simulink model "onboard_matlab"  (Simulink 8.1)
settings: Solver=FixedStepDiscrete  SolverMode=MultiTasking  StartTime=0.0  StopTime=30  FixedStep=Sampletime.Onboard  RelTol=1e-3
PreLoadFcn:
  | InitOnboardMatlab_bus;
InitFcn:
  | InitOnboardMatlab;
undefined symbols (not defined in the file or in its folder): DiscIntNeverNeededParam, Sampletime, uart_up_p_01, uart_up_p_02, uart_up_p_10, uart_up_p_11, uart_up_p_12, uart_up_p_13, uart_up_p_14
libraries: simulink x5
CloseFcn:
  | rtwprivate ssgencode ModelCloseRequest onboard_matlab
settings Model: MinMaxOverflowLogging=MinMaxAndOverflow  Creator=Holzapfel  LastModifiedBy=Javid  TunableVars=uart_up_p_01,uart_up_p_02,uart_up_p_03,uart_up_p_04,uart_up_p_05,uart_up_p_06,uart_up_p_07,uart_up_p_08,uart_up_p_09,uart_up_p_10,uart_up_p_11,uart_up_p_12,uart_up_p_13,uart_up_p_14,uart_up_p_15,uart_up_p_16,uart_up_p_17,uart_up_p_18,uart_up_p_19,uart_up_p_20,uart_up_p_21,uart_up_p_22,uart_up_p_23,uart_up_p_24,uart_up_p_25,uart_up_p_26,uart_up_p_27,uart_up_p_28,uart_up_p_29,uart_up_p_30,uart_up_p_31,uart_up_p_32,uart_up_p_33,uart_up_p_34,uart_up_p_35,uart_up_p_36,uart_up_p_37,uart_up_p_38,uart_up_p_39,uart_up_p_40  TunableVarsStorageClass=ImportedExtern,ImportedExtern,ImportedExtern,ImportedExtern,ImportedExtern,ImportedExtern,ImportedExtern,ImportedExtern,ImportedExtern,ImportedExtern,ImportedExtern,ImportedExtern,ImportedExtern,ImportedExtern,ImportedExtern,ImportedExtern,ImportedExtern,ImportedExtern,ImportedExtern,ImportedExtern,ImportedExtern,ImportedExtern,ImportedExtern,ImportedExtern,ImportedExtern,ImportedExtern,ImportedExtern,ImportedExtern,ImportedExtern,ImportedExtern,ImportedExtern,ImportedExtern,ImportedExtern,ImportedExtern,ImportedExtern,ImportedExtern,ImportedExtern,ImportedExtern,ImportedExtern,ImportedExtern  TunableVarsTypeQualifier=,,,,,,,,,,,,,,,,,,,,,,,,,,,,,,,,,,,,,,,
settings DataIOCC: LimitDataPoints=off  SaveOutput=off  SignalLogging=off  DSMLogging=off  SaveTime=off
settings OptimizationCC: InlineParams=on  InlineInvariantSignals=on  EnableMemcpy=off  StateBitsets=on  DataBitsets=on  UseTempVars=on  ZeroExternalMemoryAtStartup=off  ZeroInternalMemoryAtStartup=off  NoFixptDivByZeroProtection=on  EfficientFloat2IntCast=on  OptimizeModelRefInitCode=on  LifeSpan=1  SimCompilerOptimization=On
settings DebuggingCC: ConsistencyChecking=error  ArrayBoundsChecking=error  SignalInfNanChecking=error  SignalRangeChecking=error  ReadBeforeWriteMsg=EnableAllAsError  WriteAfterWriteMsg=EnableAllAsError  WriteAfterReadMsg=EnableAllAsError  AlgebraicLoopMsg=error  ArtificialAlgebraicLoopMsg=error  SaveWithDisabledLinksMsg=error  SaveWithParameterizedLinksMsg=error  CheckExecutionContextPreStartOutputMsg=on  CheckExecutionContextRuntimeOutputMsg=on  BlockPriorityViolationMsg=error  MinStepSizeMsg=error  TimeAdjustmentMsg=warning  SolverPrmCheckMsg=error  InheritedTsInSrcMsg=error  DiscreteInheritContinuousMsg=error  SingleTaskRateTransMsg=error  TasksWithSamePriorityMsg=error  SigSpecEnsureSampleTimeMsg=error  CheckMatrixSingularityMsg=error  IntegerOverflowMsg=error  ParameterUnderflowMsg=warning  ParameterTunabilityLossMsg=error  UnderSpecifiedDataTypeMsg=error  UnnecessaryDatatypeConvMsg=warning  VectorMatrixConversionMsg=error  SignalLabelMismatchMsg=error  UnconnectedInputMsg=error  UnconnectedOutputMsg=error  UnconnectedLineMsg=error  SFcnCompatibilityMsg=error  UniqueDataStoreMsg=error  BusObjectLabelMismatch=error  RootOutportRequireBusObject=error  ModelReferenceIOMsg=error  ModelReferenceVersionMismatchMessage=error  ModelReferenceIOMismatchMessage=error  ModelReferenceCSMismatchMessage=error  UnknownTsInhSupMsg=error  ModelReferenceDataLoggingMessage=error  StrictBusMsg=ErrorOnBusTreatedAsVector  LoggingUnavailableSignals=none
settings HardwareCC: ProdLargestAtomicInteger=Long  ProdLargestAtomicFloat=Float  ProdIntDivRoundTo=Zero  ProdEndianess=LittleEndian  ProdHWDeviceType=ARM Compatible->ARM 7  TargetEndianess=LittleEndian  TargetHWDeviceType=ARM Compatible->ARM 7
settings SFSimCC: SimParseCustomCode=off
settings RTWCC: SystemTargetFile=ert.tlc  GenCodeOnly=on  MakeCommand=make_rtw optimized_fixed_point=1  GenerateMakefile=off  TemplateMakefile=ert_default_tmf  Description=Real-Time Workshop Embedded Coder (auto configures for optimized fixed-point code)  GenerateReport=on  ProcessScript=ert_make_rtw_hook  IncludeHyperlinkInReport=on  LaunchReport=on  GenerateTraceInfo=on
settings RTWCC: CustomHeaderCode=|
  | #undef a
  | #undef b
settings CodeAppCC: IgnoreCustomStorageClasses=off  CustomSymbolStrType=$N$R$M  InternalIdentifier=Classic
settings ERTTargetCC: CodeReplacementLibrary=ANSI_C  MultiwordLength=2048  GenerateSampleERTMain=on  IncludeMdlTerminateFcn=off  SuppressErrorStatus=on  SupportNonFinite=off  SupportComplex=off  PurelyIntegerCode=on  ExtModeTransport=1  ExtModeMexFile=ext_serial_win32_comm  InlinedParameterPlacement=NonHierarchical  ERTCustomFileTemplate=file_process.tlc  ConvertIfToSwitch=off  SuppressUnreachableDefaultCases=off

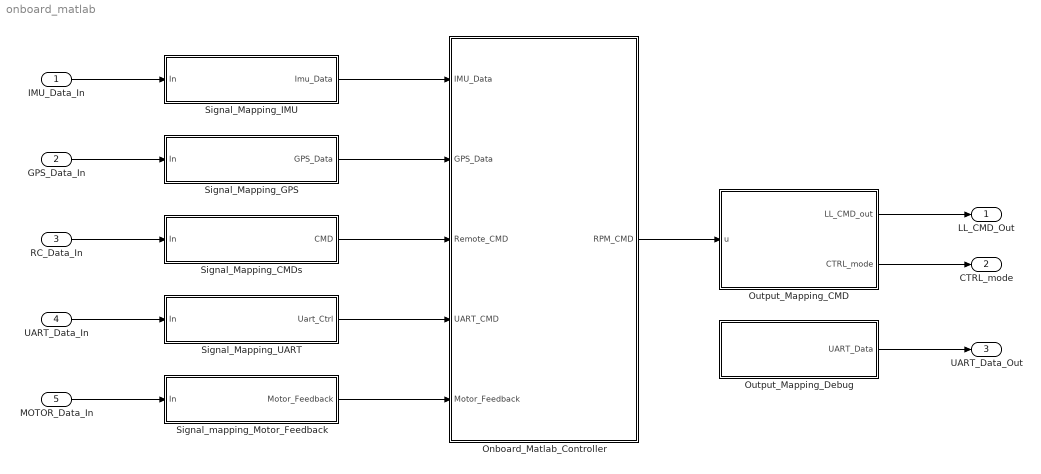
== system onboard_matlab ==
  IMU_Data_In : Inport  OutMin=-2^31  OutMax=2^31-1  OutDataTypeStr=Bus: IMU_DATA_IN  SampleTime=Sampletime.Onboard  BusOutputAsStruct=on
  GPS_Data_In : Inport  Port=2  OutMin=-2^31  OutMax=2^31-1  OutDataTypeStr=Bus: GPS_DATA_IN  SampleTime=Sampletime.Onboard  BusOutputAsStruct=on
  RC_Data_In : Inport  Port=3  OutMin=-2^15  OutMax=2^15-1  OutDataTypeStr=Bus: RC_DATA_IN  SampleTime=Sampletime.Onboard  BusOutputAsStruct=on
  UART_Data_In : Inport  Port=4  OutMin=-2^15  OutMax=2^15-1  OutDataTypeStr=Bus: UART_DATA_IN  SampleTime=Sampletime.Onboard  BusOutputAsStruct=on
  MOTOR_Data_In : Inport  Port=5  OutMin=0  OutMax=200  OutDataTypeStr=Bus: MOTOR_DATA_IN  SampleTime=Sampletime.Onboard  BusOutputAsStruct=on
  Onboard_Matlab_Controller : Subsystem  MinMaxOverflowLogging=MinMaxAndOverflow
  Output_Mapping_CMD : Subsystem
  Output_Mapping_Debug : Subsystem
  Signal_Mapping_CMDs : Subsystem
  Signal_Mapping_GPS : Subsystem
  Signal_Mapping_IMU : Subsystem
  Signal_Mapping_UART : Subsystem
  Signal_mapping_Motor_Feedback : Subsystem
  LL_CMD_Out : Outport  OutDataTypeStr=Bus: LL_CMD_OUT  SampleTime=Sampletime.Onboard  BusOutputAsStruct=on
  CTRL_mode : Outport  Port=2  OutDataTypeStr=Bus: CTRL_MODE  SampleTime=Sampletime.Onboard  BusOutputAsStruct=on
  UART_Data_Out : Outport  Port=3  OutDataTypeStr=Bus: UART_DATA_OUT  SampleTime=Sampletime.Onboard  BusOutputAsStruct=on
  wires:
  RC_Data_In/1 -> Signal_Mapping_CMDs/1(In)
  Signal_Mapping_CMDs/1(CMD) -> Onboard_Matlab_Controller/3(Remote_CMD)
  Onboard_Matlab_Controller/1(RPM_CMD) -> Output_Mapping_CMD/1(u)
  Output_Mapping_CMD/1(LL_CMD_out) -> LL_CMD_Out/1
  IMU_Data_In/1 -> Signal_Mapping_IMU/1(In)
  Signal_Mapping_IMU/1(Imu_Data) -> Onboard_Matlab_Controller/1(IMU_Data)
  GPS_Data_In/1 -> Signal_Mapping_GPS/1(In)
  Signal_Mapping_GPS/1(GPS_Data) -> Onboard_Matlab_Controller/2(GPS_Data)
  UART_Data_In/1 -> Signal_Mapping_UART/1(In)
  Signal_Mapping_UART/1(Uart_Ctrl) -> Onboard_Matlab_Controller/4(UART_CMD)
  Output_Mapping_Debug/1(UART_Data) -> UART_Data_Out/1
  MOTOR_Data_In/1 -> Signal_mapping_Motor_Feedback/1(In)
  Signal_mapping_Motor_Feedback/1(Motor_Feedback) -> Onboard_Matlab_Controller/5(Motor_Feedback)
  Output_Mapping_CMD/2(CTRL_mode) -> CTRL_mode/1

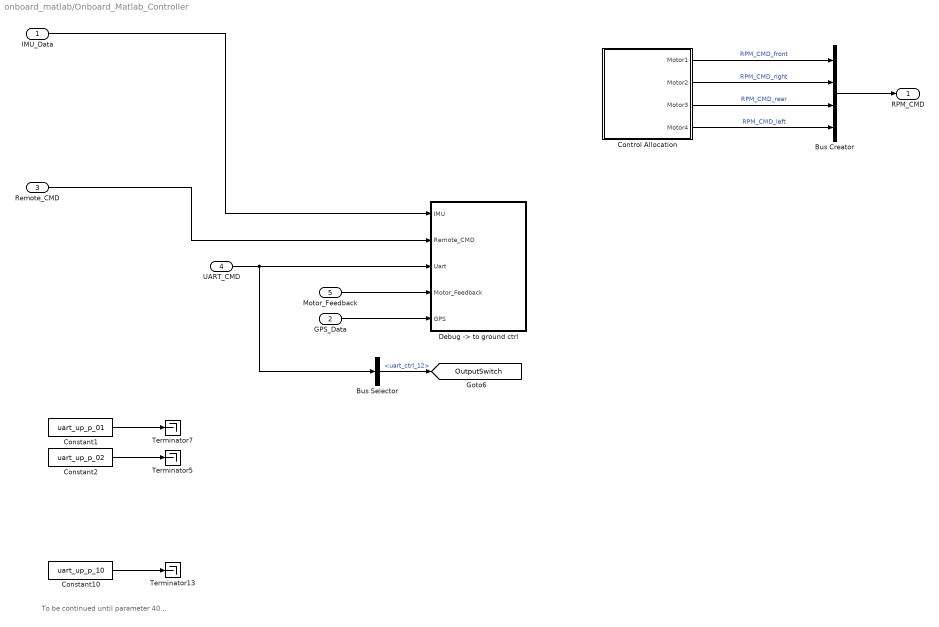
== system onboard_matlab/Onboard_Matlab_Controller ==
  note: To be continued until parameter 40...
  IMU_Data : Inport
  GPS_Data : Inport  Port=2
  Remote_CMD : Inport  Port=3
  UART_CMD : Inport  Port=4
  Motor_Feedback : Inport  Port=5
  Bus Creator : BusCreator
  Bus Selector : BusSelector  OutputSignals=uart_ctrl_12
  Constant1 : Constant  Value=uart_up_p_01  OutMin=-2^15  OutMax=2^15-1  OutDataTypeStr=fixdt(1,32,16)
  Constant10 : Constant  Value=uart_up_p_10  OutMin=-2^15  OutMax=2^15-1  OutDataTypeStr=fixdt(1,32,16)
  Constant2 : Constant  Value=uart_up_p_02  OutMin=-2^15  OutMax=2^15-1  OutDataTypeStr=fixdt(1,32,16)
  Control Allocation : Subsystem
  "Debug -> to ground ctrl" : Subsystem
  Terminator13 : Terminator
  Terminator5 : Terminator
  Terminator7 : Terminator
  RPM_CMD : Outport
  tag scope: OutputSwitch=global
  wires:
  Control Allocation/4(Motor4) -> Bus Creator/4  "RPM_CMD_left"
  Control Allocation/3(Motor3) -> Bus Creator/3  "RPM_CMD_rear"
  Control Allocation/2(Motor2) -> Bus Creator/2  "RPM_CMD_right"
  Control Allocation/1(Motor1) -> Bus Creator/1  "RPM_CMD_front"
  Bus Creator/1 -> RPM_CMD/1
  Remote_CMD/1 -> "Debug -> to ground ctrl"/2(Remote_CMD)
  IMU_Data/1 -> "Debug -> to ground ctrl"/1(IMU)
  UART_CMD/1 -> Bus Selector/1, "Debug -> to ground ctrl"/3(Uart)
  Constant2/1 -> Terminator5/1
  Constant10/1 -> Terminator13/1
  Constant1/1 -> Terminator7/1
  Bus Selector/1 -> [OutputSwitch]  "<uart_ctrl_12>"
  Motor_Feedback/1 -> "Debug -> to ground ctrl"/4(Motor_Feedback)
  GPS_Data/1 -> "Debug -> to ground ctrl"/5(GPS)

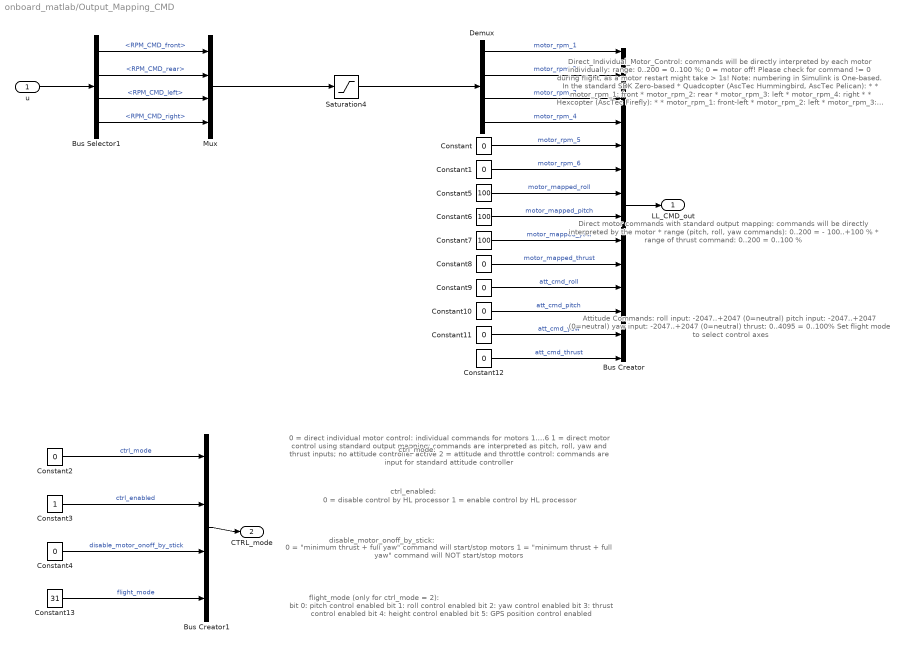
== system onboard_matlab/Output_Mapping_CMD ==
  note: 0 = direct individual motor control: individual commands for motors 1....6
      | 1 = direct motor control using standard output mapping: commands are interpreted as pitch, roll, yaw and thrust inputs; no attitude controller active
      | 2 = attitude and throttle control: commands are input for standard attitude controller
  note: ctrl_mode:
  note: 0 = disable control by HL processor
      | 1 = enable control by HL processor
  note: ctrl_enabled:
  note: 0 = "minimum thrust + full yaw" command will start/stop motors
      | 1 = "minimum thrust + full yaw" command will NOT start/stop motors
  note: disable_motor_onoff_by_stick:
  note: bit 0: pitch control enabled
      | 							bit 1: roll control enabled
      | 							bit 2: yaw control enabled
      | 							bit 3: thrust control enabled
      | 							bit 4: height control enabled
      | 							bit 5: GPS position control enabled
  note: flight_mode (only for ctrl_mode = 2):
  note: Direct_Individual_Motor_Control:
      | commands will be directly interpreted by each motor individually: range: 0..200 = 0..100 %; 0 = motor off! Please check for command != 0 during flight, as a motor restart might take > 1s!
      | Note: numbering in Simulink is One-based. In the standard SDK Zero-based
      |
      | 	 * Quadcopter (AscTec Hummingbird, AscTec Pelican):	 *
      | 	 * motor_rpm_1: front
      | 	 * motor_rpm_2: rear
      | 	 * motor_rpm_3: left
      | 	 * motor_rpm_4: right
      | 	 *
      | 	 * Hexcopter (AscTec Firefly):	 *
      | 	 * motor_rpm_1: front-left
      | 	 * motor_rpm_2: left
      | 	 * motor_rpm_3: rear-left
      | 	 * motor_rpm_4: rear-right
      | 	 * motor_rpm_5: right
      | 	 * motor_rpm_6: front-right
  note: Attitude Commands:
      | roll input: -2047..+2047	(0=neutral)
      | pitch input: -2047..+2047 (0=neutral)
      | yaw input: -2047..+2047	(0=neutral)
      | thrust: 0..4095 = 0..100%
      |
      | Set flight mode to select control axes
  note: Direct motor commands with standard output mapping:
      | commands will be directly interpreted by the motor
      | 	 * range (pitch, roll, yaw commands): 0..200 = - 100..+100 %
      | 	 * range of thrust command: 0..200 = 0..100 %
  u : Inport
  Bus Creator : BusCreator  Inputs=14
  Bus Creator1 : BusCreator
  Bus Selector1 : BusSelector  OutputSignals=RPM_CMD_front,RPM_CMD_rear,RPM_CMD_left,RPM_CMD_right
  Constant{,1,8..12} (7 alike) : Constant  Value=0  OutDataTypeStr=int16
  Constant13 : Constant  Value=31  OutDataTypeStr=int16
  Constant2 : Constant  Value=0  OutDataTypeStr=uint8
  Constant3 : Constant  OutDataTypeStr=uint8
  Constant4 : Constant  Value=0  OutDataTypeStr=uint8
  Constant5 : Constant  Value=100  OutDataTypeStr=int16
  Constant6 : Constant  Value=100  OutDataTypeStr=int16
  Constant7 : Constant  Value=100  OutDataTypeStr=int16
  Demux : Demux
  Mux : Mux
  Saturation4 : Saturate  UpperLimit=200  LowerLimit=1  OutDataTypeStr=int16  RndMeth=Zero
  LL_CMD_out : Outport
  CTRL_mode : Outport  Port=2
  wires:
  u/1 -> Bus Selector1/1
  Mux/1 -> Saturation4/1
  Bus Creator/1 -> LL_CMD_out/1
  Saturation4/1 -> Demux/1
  Demux/1 -> Bus Creator/1  "motor_rpm_1"
  Demux/2 -> Bus Creator/2  "motor_rpm_2"
  Demux/3 -> Bus Creator/3  "motor_rpm_3"
  Demux/4 -> Bus Creator/4  "motor_rpm_4"
  Constant/1 -> Bus Creator/5  "motor_rpm_5"
  Constant1/1 -> Bus Creator/6  "motor_rpm_6"
  Bus Selector1/1 -> Mux/1  "<RPM_CMD_front>"
  Bus Selector1/2 -> Mux/2  "<RPM_CMD_rear>"
  Bus Selector1/3 -> Mux/3  "<RPM_CMD_left>"
  Bus Selector1/4 -> Mux/4  "<RPM_CMD_right>"
  Constant2/1 -> Bus Creator1/1  "ctrl_mode"
  Constant3/1 -> Bus Creator1/2  "ctrl_enabled"
  Constant4/1 -> Bus Creator1/3  "disable_motor_onoff_by_stick"
  Bus Creator1/1 -> CTRL_mode/1
  Constant5/1 -> Bus Creator/7  "motor_mapped_roll"
  Constant6/1 -> Bus Creator/8  "motor_mapped_pitch"
  Constant7/1 -> Bus Creator/9  "motor_mapped_yaw"
  Constant8/1 -> Bus Creator/10  "motor_mapped_thrust"
  Constant9/1 -> Bus Creator/11  "att_cmd_roll"
  Constant10/1 -> Bus Creator/12  "att_cmd_pitch"
  Constant11/1 -> Bus Creator/13  "att_cmd_yaw"
  Constant12/1 -> Bus Creator/14  "att_cmd_thrust"
  Constant13/1 -> Bus Creator1/4  "flight_mode"

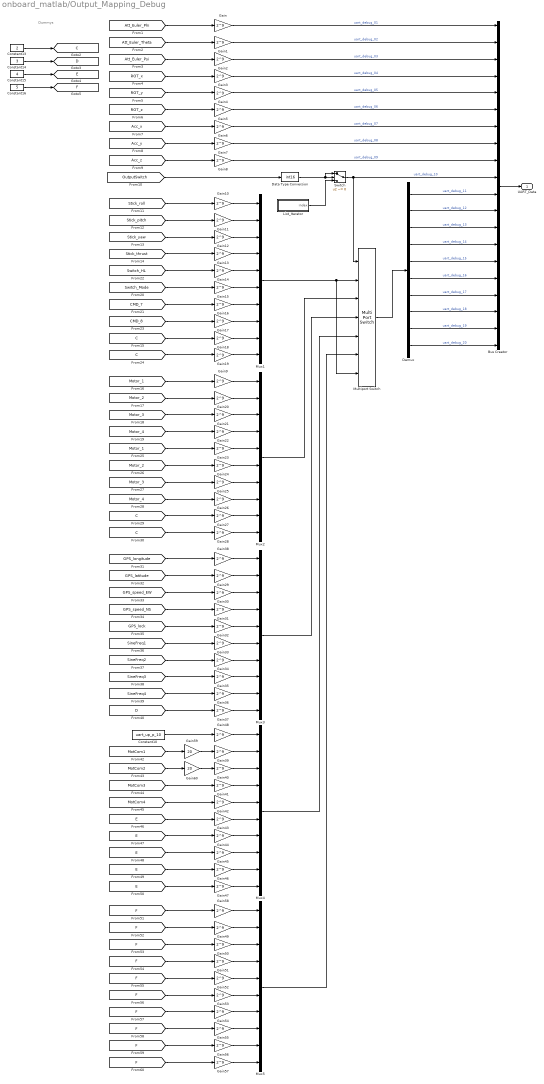
== system onboard_matlab/Output_Mapping_Debug ==
  note: Dummys
  Bus Creator : BusCreator  Inputs=20
  Constant10 : Constant  Value=uart_up_p_10  OutMin=-2^15  OutMax=2^15-1  OutDataTypeStr=fixdt(1,32,16)
  Constant13 : Constant  Value=2  OutMin=-64  OutMax=63  OutDataTypeStr=fixdt(1,16,9)
  Constant14 : Constant  Value=3  OutMin=-64  OutMax=63  OutDataTypeStr=fixdt(1,16,9)
  Constant15 : Constant  Value=4  OutMin=-64  OutMax=63  OutDataTypeStr=fixdt(1,16,9)
  Constant16 : Constant  Value=5  OutMin=-64  OutMax=63  OutDataTypeStr=fixdt(1,16,9)
  Data Type Conversion : DataTypeConversion  OutDataTypeStr=int16
  Demux : Demux  Outputs=10
  Gain{,1..58} (59 alike) : Gain  Gain=2^9  OutDataTypeStr=int16  SaturateOnIntegerOverflow=on
  Gain59 : Gain  Gain=20  OutDataTypeStr=fixdt(1,32,16)  SaturateOnIntegerOverflow=on
  Gain60 : Gain  Gain=20  OutDataTypeStr=fixdt(1,32,16)  SaturateOnIntegerOverflow=on
  List_Iterator : Subsystem  mask(Iterator){list=[1;2;3;4;5;], dec=1/Sampletime.Onboard/50}
      mask prompts: list "List of indices to iterate"; dec "Rate decimation"
      mask help: Outputs a sequence of numbers specified by a list of arbitrary length. The rate can be decimated by an integer factor.
  Multiport Switch : MultiPortSwitch  Inputs=5  DataPortForDefault=Additional data port  DiagnosticForDefault=None  InputSameDT=on
  Mux{1..5} (5 alike) : Mux  Inputs=10
  Switch : Switch  Criteria=u2 ~= 0
  UART_Data : Outport
  tag scope: C=global, D=global, E=global, F=global
  wires:
  Constant16/1 -> [F]
  Constant15/1 -> [E]
  Constant14/1 -> [D]
  Constant13/1 -> [C]
  Data Type Conversion/1 -> Switch/1, Switch/2
  Switch/1 -> Bus Creator/10, Multiport Switch/1  "uart_debug_10"
  List_Iterator/1(index) -> Switch/3
  [OutputSwitch] -> Data Type Conversion/1
  Mux5/1 -> Multiport Switch/6
  Gain57/1 -> Mux5/10
  Gain56/1 -> Mux5/9
  Gain55/1 -> Mux5/8
  Gain54/1 -> Mux5/7
  Gain53/1 -> Mux5/6
  Gain52/1 -> Mux5/5
  Gain51/1 -> Mux5/4
  Gain50/1 -> Mux5/3
  Gain49/1 -> Mux5/2
  Gain58/1 -> Mux5/1
  [F] -> Gain57/1
  [F] -> Gain56/1
  [F] -> Gain55/1
  [F] -> Gain54/1
  [F] -> Gain53/1
  [F] -> Gain52/1
  [F] -> Gain51/1
  [F] -> Gain50/1
  [F] -> Gain49/1
  [F] -> Gain58/1
  Multiport Switch/1 -> Demux/1
  Mux4/1 -> Multiport Switch/5
  Gain47/1 -> Mux4/10
  Gain46/1 -> Mux4/9
  Gain45/1 -> Mux4/8
  Gain44/1 -> Mux4/7
  Gain43/1 -> Mux4/6
  Gain42/1 -> Mux4/5
  Gain41/1 -> Mux4/4
  Gain40/1 -> Mux4/3
  Gain39/1 -> Mux4/2
  Gain48/1 -> Mux4/1
  [E] -> Gain47/1
  [E] -> Gain46/1
  [E] -> Gain45/1
  [E] -> Gain44/1
  [E] -> Gain43/1
  [MotCom4] -> Gain42/1
  [MotCom3] -> Gain41/1
  [MotCom2] -> Gain60/1
  [MotCom1] -> Gain59/1
  Constant10/1 -> Gain48/1
  Mux3/1 -> Multiport Switch/4
  Gain37/1 -> Mux3/10
  Gain36/1 -> Mux3/9
  Gain35/1 -> Mux3/8
  Gain34/1 -> Mux3/7
  Gain33/1 -> Mux3/6
  Gain32/1 -> Mux3/5
  Gain31/1 -> Mux3/4
  Gain30/1 -> Mux3/3
  Gain29/1 -> Mux3/2
  Gain38/1 -> Mux3/1
  [D] -> Gain37/1
  [SineFreq4] -> Gain36/1
  [SineFreq3] -> Gain35/1
  [SineFreq2] -> Gain34/1
  [SineFreq1] -> Gain33/1
  [GPS_lock] -> Gain32/1
  [GPS_speed_NS] -> Gain31/1
  [GPS_speed_EW] -> Gain30/1
  [GPS_latitude] -> Gain29/1
  [GPS_longitude] -> Gain38/1
  Mux2/1 -> Multiport Switch/3
  Gain28/1 -> Mux2/10
  Gain27/1 -> Mux2/9
  Gain26/1 -> Mux2/8
  Gain25/1 -> Mux2/7
  Gain24/1 -> Mux2/6
  Gain23/1 -> Mux2/5
  Gain22/1 -> Mux2/4
  Gain21/1 -> Mux2/3
  Gain20/1 -> Mux2/2
  Gain9/1 -> Mux2/1
  [C] -> Gain28/1
  [C] -> Gain27/1
  [Motor_4] -> Gain26/1
  [Motor_3] -> Gain25/1
  [Motor_2] -> Gain24/1
  [Motor_1] -> Gain23/1
  [Motor_4] -> Gain22/1
  [Motor_3] -> Gain21/1
  [Motor_2] -> Gain20/1
  [Motor_1] -> Gain9/1
  Mux1/1 -> Multiport Switch/7, Multiport Switch/2
  Gain19/1 -> Mux1/10
  Gain18/1 -> Mux1/9
  Gain17/1 -> Mux1/8
  Gain16/1 -> Mux1/7
  Gain15/1 -> Mux1/6
  Gain14/1 -> Mux1/5
  Gain13/1 -> Mux1/4
  Gain12/1 -> Mux1/3
  Gain11/1 -> Mux1/2
  Gain10/1 -> Mux1/1
  [C] -> Gain19/1
  [C] -> Gain18/1
  [CMD_8] -> Gain17/1
  [CMD_7] -> Gain16/1
  [Switch_Mode] -> Gain15/1
  [Switch_HL] -> Gain14/1
  [Stick_thrust] -> Gain13/1
  [Stick_yaw] -> Gain12/1
  [Stick_pitch] -> Gain11/1
  [Stick_roll] -> Gain10/1
  [Acc_z] -> Gain8/1
  [Acc_y] -> Gain7/1
  [Acc_x] -> Gain6/1
  [ROT_z] -> Gain5/1
  [ROT_y] -> Gain4/1
  [ROT_x] -> Gain3/1
  [Att_Euler_Psi] -> Gain2/1
  [Att_Euler_Theta] -> Gain1/1
  [Att_Euler_Phi] -> Gain/1
  Demux/10 -> Bus Creator/20  "uart_debug_20"
  Demux/9 -> Bus Creator/19  "uart_debug_19"
  Demux/8 -> Bus Creator/18  "uart_debug_18"
  Demux/7 -> Bus Creator/17  "uart_debug_17"
  Demux/6 -> Bus Creator/16  "uart_debug_16"
  Demux/5 -> Bus Creator/15  "uart_debug_15"
  Demux/4 -> Bus Creator/14  "uart_debug_14"
  Demux/3 -> Bus Creator/13  "uart_debug_13"
  Demux/2 -> Bus Creator/12  "uart_debug_12"
  Demux/1 -> Bus Creator/11  "uart_debug_11"
  Gain8/1 -> Bus Creator/9  "uart_debug_09"
  Gain7/1 -> Bus Creator/8  "uart_debug_08"
  Gain6/1 -> Bus Creator/7  "uart_debug_07"
  Gain5/1 -> Bus Creator/6  "uart_debug_06"
  Gain4/1 -> Bus Creator/5  "uart_debug_05"
  Gain3/1 -> Bus Creator/4  "uart_debug_04"
  Gain2/1 -> Bus Creator/3  "uart_debug_03"
  Gain1/1 -> Bus Creator/2  "uart_debug_02"
  Gain/1 -> Bus Creator/1  "uart_debug_01"
  Bus Creator/1 -> UART_Data/1
  Gain60/1 -> Gain40/1
  Gain59/1 -> Gain39/1

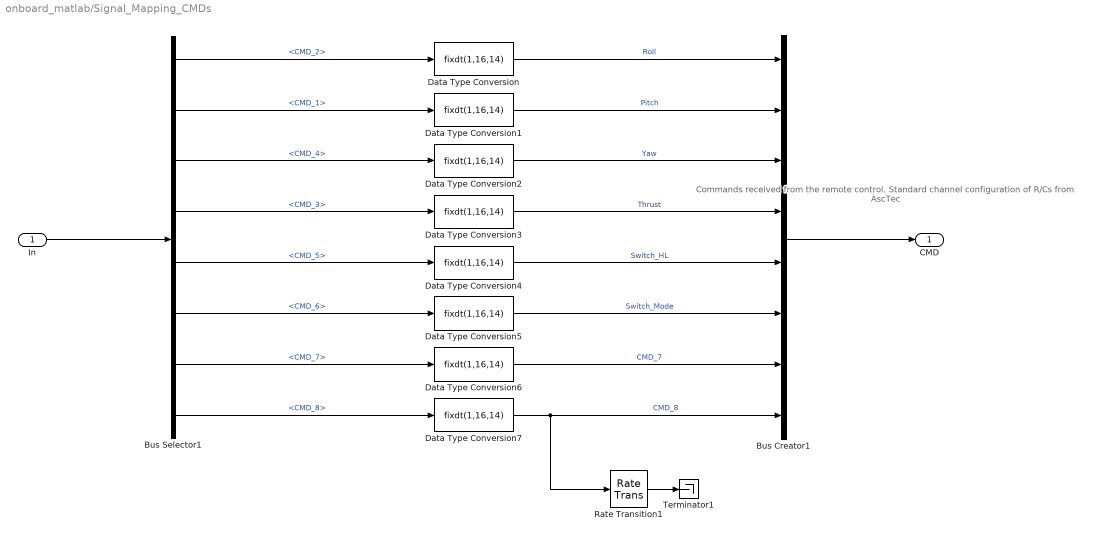
== system onboard_matlab/Signal_Mapping_CMDs ==
  note: Commands received from the remote control.
      | Standard channel configuration
      | of R/Cs from AscTec
  In : Inport
  Bus Creator1 : BusCreator  Inputs=8
  Bus Selector1 : BusSelector  OutputSignals=CMD_2,CMD_1,CMD_4,CMD_3,CMD_5,CMD_6,CMD_7,CMD_8
  Data Type Conversion{,1..7} (8 alike) : DataTypeConversion  OutDataTypeStr=fixdt(1,16,14)  ConvertRealWorld=Stored Integer (SI)  RndMeth=Simplest
  Rate Transition1 : RateTransition  Integrity=off  Deterministic=off  OutPortSampleTimeOpt=Multiple of input port sample time  OutPortSampleTimeMultiple=2  OutPortSampleTime=0.002
  Terminator1 : Terminator
  CMD : Outport
  wires:
  In/1 -> Bus Selector1/1
  Bus Selector1/1 -> Data Type Conversion/1  "<CMD_2>"
  Bus Selector1/2 -> Data Type Conversion1/1  "<CMD_1>"
  Bus Selector1/3 -> Data Type Conversion2/1  "<CMD_4>"
  Bus Selector1/4 -> Data Type Conversion3/1  "<CMD_3>"
  Bus Selector1/5 -> Data Type Conversion4/1  "<CMD_5>"
  Bus Selector1/6 -> Data Type Conversion5/1  "<CMD_6>"
  Bus Selector1/7 -> Data Type Conversion6/1  "<CMD_7>"
  Bus Selector1/8 -> Data Type Conversion7/1  "<CMD_8>"
  Data Type Conversion/1 -> Bus Creator1/1  "Roll"
  Data Type Conversion1/1 -> Bus Creator1/2  "Pitch"
  Data Type Conversion2/1 -> Bus Creator1/3  "Yaw"
  Data Type Conversion3/1 -> Bus Creator1/4  "Thrust"
  Data Type Conversion4/1 -> Bus Creator1/5  "Switch_HL"
  Data Type Conversion5/1 -> Bus Creator1/6  "Switch_Mode"
  Data Type Conversion6/1 -> Bus Creator1/7  "CMD_7"
  Data Type Conversion7/1 -> Bus Creator1/8, Rate Transition1/1  "CMD_8"
  Bus Creator1/1 -> CMD/1
  Rate Transition1/1 -> Terminator1/1

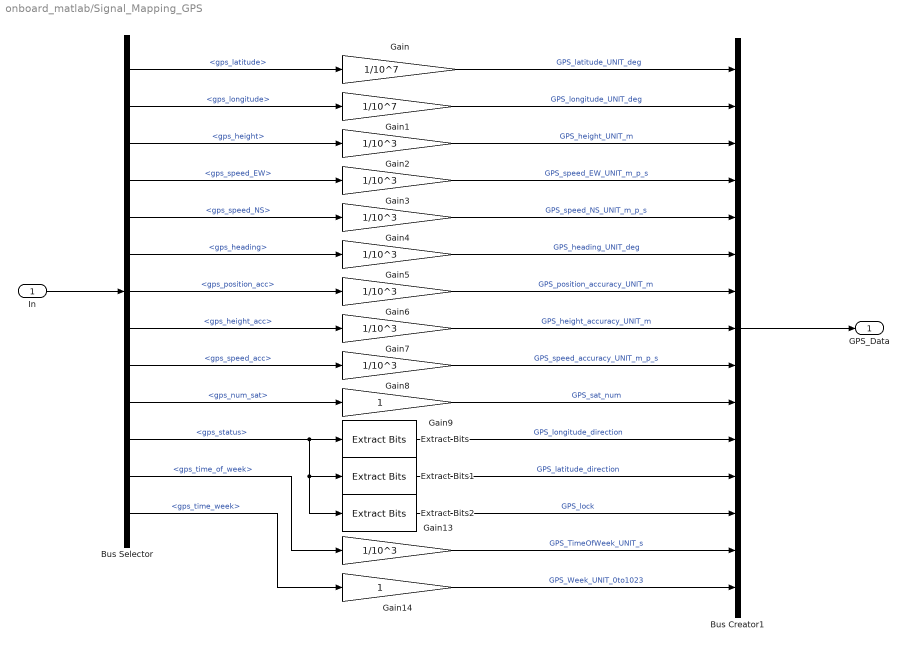
== system onboard_matlab/Signal_Mapping_GPS ==
  In : Inport
  Bus Creator1 : BusCreator  Inputs=15
  Bus Selector : BusSelector  OutputSignals=gps_latitude,gps_longitude,gps_height,gps_speed_EW,gps_speed_NS,gps_heading,gps_position_acc,gps_height_acc,gps_speed_acc,gps_num_sat,gps_status,gps_time_of_week,gps_time_week
  Extract Bits : simulink/Logic and Bit Operations/Extract Bits  bitsToExtract=Range of bits  numBits=8  bitIdxRange=2  outScalingMode=Treat bit field as an integer
  Extract Bits1 : simulink/Logic and Bit Operations/Extract Bits  bitsToExtract=Range of bits  numBits=8  bitIdxRange=1  outScalingMode=Treat bit field as an integer
  Extract Bits2 : simulink/Logic and Bit Operations/Extract Bits  bitsToExtract=Range of bits  numBits=8  bitIdxRange=0  outScalingMode=Treat bit field as an integer
  Gain : Gain  Gain=1/10^7  OutMin=-90  OutMax=90  OutDataTypeStr=fixdt(1,32,24)  RndMeth=Zero  SaturateOnIntegerOverflow=on  LockScale=on
  Gain1 : Gain  Gain=1/10^7  OutMin=-180  OutMax=180  OutDataTypeStr=fixdt(1,32,23)  RndMeth=Zero  SaturateOnIntegerOverflow=on  LockScale=on
  Gain13 : Gain  Gain=1/10^3  OutDataTypeStr=fixdt(0,32,10)  RndMeth=Zero  SaturateOnIntegerOverflow=on  LockScale=on
  Gain14 : Gain  OutDataTypeStr=uint16  RndMeth=Zero  SaturateOnIntegerOverflow=on  LockScale=on
  Gain2 : Gain  Gain=1/10^3  OutDataTypeStr=fixdt(1,32,10)  RndMeth=Zero  SaturateOnIntegerOverflow=on  LockScale=on
  Gain3 : Gain  Gain=1/10^3  OutDataTypeStr=fixdt(1,32,10)  RndMeth=Zero  SaturateOnIntegerOverflow=on  LockScale=on
  Gain4 : Gain  Gain=1/10^3  OutDataTypeStr=fixdt(1,32,10)  RndMeth=Zero  SaturateOnIntegerOverflow=on  LockScale=on
  Gain5 : Gain  Gain=1/10^3  OutMin=0  OutMax=360  OutDataTypeStr=fixdt(1,32,22)  RndMeth=Zero  SaturateOnIntegerOverflow=on  LockScale=on
  Gain6 : Gain  Gain=1/10^3  OutMin=0  OutMax=100  OutDataTypeStr=fixdt(1,16,8)  RndMeth=Zero  SaturateOnIntegerOverflow=on  LockScale=on
  Gain7 : Gain  Gain=1/10^3  OutMin=0  OutMax=100  OutDataTypeStr=fixdt(1,16,8)  RndMeth=Zero  SaturateOnIntegerOverflow=on  LockScale=on
  Gain8 : Gain  Gain=1/10^3  OutMin=0  OutMax=100  OutDataTypeStr=fixdt(1,16,8)  RndMeth=Zero  SaturateOnIntegerOverflow=on  LockScale=on
  Gain9 : Gain  OutDataTypeStr=uint8  RndMeth=Zero  SaturateOnIntegerOverflow=on  LockScale=on
  GPS_Data : Outport
  wires:
  In/1 -> Bus Selector/1
  Bus Creator1/1 -> GPS_Data/1
  Bus Selector/1 -> Gain/1  "<gps_latitude>"
  Bus Selector/2 -> Gain1/1  "<gps_longitude>"
  Bus Selector/3 -> Gain2/1  "<gps_height>"
  Bus Selector/4 -> Gain3/1  "<gps_speed_EW>"
  Bus Selector/5 -> Gain4/1  "<gps_speed_NS>"
  Bus Selector/6 -> Gain5/1  "<gps_heading>"
  Bus Selector/7 -> Gain6/1  "<gps_position_acc>"
  Bus Selector/8 -> Gain7/1  "<gps_height_acc>"
  Bus Selector/9 -> Gain8/1  "<gps_speed_acc>"
  Bus Selector/10 -> Gain9/1  "<gps_num_sat>"
  Gain8/1 -> Bus Creator1/9  "GPS_speed_accuracy_UNIT_m_p_s"
  Gain9/1 -> Bus Creator1/10  "GPS_sat_num"
  Gain7/1 -> Bus Creator1/8  "GPS_height_accuracy_UNIT_m"
  Gain6/1 -> Bus Creator1/7  "GPS_position_accuracy_UNIT_m"
  Gain5/1 -> Bus Creator1/6  "GPS_heading_UNIT_deg"
  Gain4/1 -> Bus Creator1/5  "GPS_speed_NS_UNIT_m_p_s"
  Gain3/1 -> Bus Creator1/4  "GPS_speed_EW_UNIT_m_p_s"
  Gain2/1 -> Bus Creator1/3  "GPS_height_UNIT_m"
  Gain1/1 -> Bus Creator1/2  "GPS_longitude_UNIT_deg"
  Gain/1 -> Bus Creator1/1  "GPS_latitude_UNIT_deg"
  Bus Selector/12 -> Gain13/1  "<gps_time_of_week>"
  Bus Selector/13 -> Gain14/1  "<gps_time_week>"
  Bus Selector/11 -> Extract Bits/1, Extract Bits1/1, Extract Bits2/1  "<gps_status>"
  Extract Bits/1 -> Bus Creator1/11  "GPS_longitude_direction"
  Extract Bits2/1 -> Bus Creator1/13  "GPS_lock"
  Extract Bits1/1 -> Bus Creator1/12  "GPS_latitude_direction"
  Gain13/1 -> Bus Creator1/14  "GPS_TimeOfWeek_UNIT_s"
  Gain14/1 -> Bus Creator1/15  "GPS_Week_UNIT_0to1023"

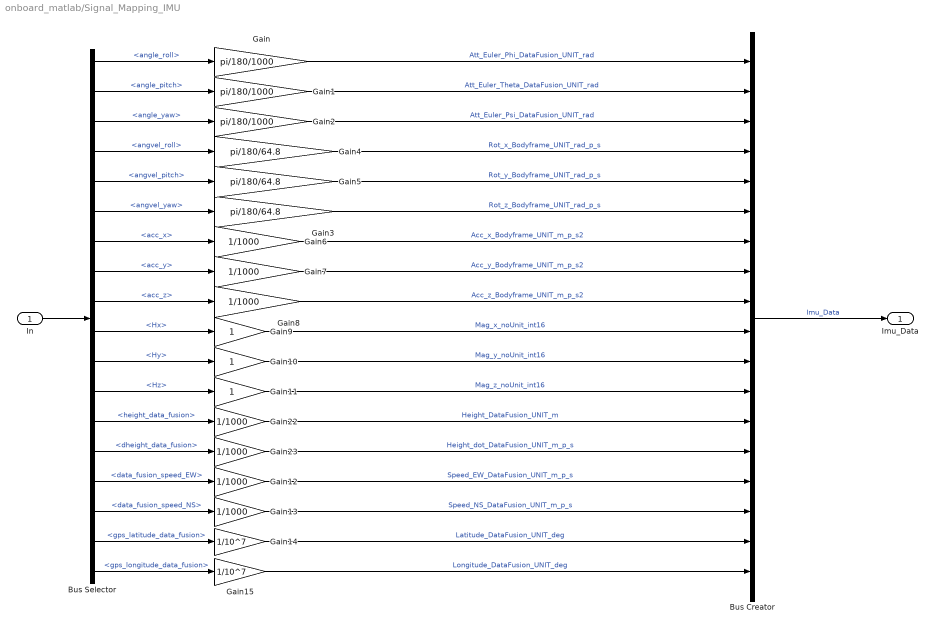
== system onboard_matlab/Signal_Mapping_IMU ==
  In : Inport
  Bus Creator : BusCreator  Inputs=18
  Bus Selector : BusSelector  OutputSignals=angle_roll,angle_pitch,angle_yaw,angvel_roll,angvel_pitch,angvel_yaw,acc_x,acc_y,acc_z,Hx,Hy,Hz,height_data_fusion,dheight_data_fusion,data_fusion_speed_EW,data_fusion_speed_NS,gps_latitude_data_fusion,gps_longitude_data_fusion
  Gain : Gain  Gain=pi/180/1000  OutMin=-0.5*pi  OutMax=0.5*pi  OutDataTypeStr=fixdt(1,16,14)  RndMeth=Simplest  LockScale=on
  Gain1 : Gain  Gain=pi/180/1000  OutMin=-0.5*pi  OutMax=0.5*pi  OutDataTypeStr=fixdt(1,16,14)  RndMeth=Simplest  LockScale=on
  Gain10 : Gain  OutDataTypeStr=int16  RndMeth=Simplest
  Gain11 : Gain  OutDataTypeStr=int16  RndMeth=Simplest
  Gain12 : Gain  Gain=1/1000  OutMin=-10  OutMax=10  OutDataTypeStr=fixdt(1,16,11)  RndMeth=Simplest  LockScale=on
  Gain13 : Gain  Gain=1/1000  OutMin=-10  OutMax=10  OutDataTypeStr=fixdt(1,16,11)  RndMeth=Simplest  LockScale=on
  Gain14 : Gain  Gain=1/10^7  OutMin=-90  OutMax=90  OutDataTypeStr=fixdt(1,32,24)  RndMeth=Zero  SaturateOnIntegerOverflow=on  LockScale=on
  Gain15 : Gain  Gain=1/10^7  OutMin=-90  OutMax=90  OutDataTypeStr=fixdt(1,32,24)  RndMeth=Zero  SaturateOnIntegerOverflow=on  LockScale=on
  Gain2 : Gain  Gain=pi/180/1000  OutMin=-0  OutMax=2*pi  OutDataTypeStr=fixdt(1,16,12)  RndMeth=Simplest  LockScale=on
  Gain22 : Gain  Gain=1/1000  OutMin=-10000  OutMax=10000  OutDataTypeStr=fixdt(1,32,17)  RndMeth=Simplest
  Gain23 : Gain  Gain=1/1000  OutMin=-10  OutMax=10  OutDataTypeStr=fixdt(1,16,11)  RndMeth=Simplest  LockScale=on
  Gain3 : Gain  Gain=pi/180/64.8  OutMin=-2*pi  OutMax=2*pi  OutDataTypeStr=fixdt(1,16,12)  RndMeth=Simplest  LockScale=on
  Gain4 : Gain  Gain=pi/180/64.8  OutMin=-2*pi  OutMax=2*pi  OutDataTypeStr=fixdt(1,16,12)  RndMeth=Simplest  LockScale=on
  Gain5 : Gain  Gain=pi/180/64.8  OutMin=-2*pi  OutMax=2*pi  OutDataTypeStr=fixdt(1,16,12)  RndMeth=Simplest  LockScale=on
  Gain6 : Gain  Gain=1/1000  OutMin=-30  OutMax=30  OutDataTypeStr=fixdt(1,16,10)  RndMeth=Simplest
  Gain7 : Gain  Gain=1/1000  OutMin=-30  OutMax=30  OutDataTypeStr=fixdt(1,16,10)  RndMeth=Simplest
  Gain8 : Gain  Gain=1/1000  OutMin=-30  OutMax=30  OutDataTypeStr=fixdt(1,16,10)  RndMeth=Simplest
  Gain9 : Gain  OutDataTypeStr=int16  RndMeth=Simplest
  Imu_Data : Outport
  wires:
  In/1 -> Bus Selector/1
  Bus Selector/1 -> Gain/1  "<angle_roll>"
  Gain/1 -> Bus Creator/1  "Att_Euler_Phi_DataFusion_UNIT_rad"
  Gain1/1 -> Bus Creator/2  "Att_Euler_Theta_DataFusion_UNIT_rad"
  Gain2/1 -> Bus Creator/3  "Att_Euler_Psi_DataFusion_UNIT_rad"
  Bus Selector/2 -> Gain1/1  "<angle_pitch>"
  Bus Selector/3 -> Gain2/1  "<angle_yaw>"
  Bus Selector/5 -> Gain5/1  "<angvel_pitch>"
  Bus Selector/4 -> Gain4/1  "<angvel_roll>"
  Gain4/1 -> Bus Creator/4  "Rot_x_Bodyframe_UNIT_rad_p_s"
  Gain5/1 -> Bus Creator/5  "Rot_y_Bodyframe_UNIT_rad_p_s"
  Bus Selector/6 -> Gain3/1  "<angvel_yaw>"
  Gain3/1 -> Bus Creator/6  "Rot_z_Bodyframe_UNIT_rad_p_s"
  Bus Selector/7 -> Gain6/1  "<acc_x>"
  Gain6/1 -> Bus Creator/7  "Acc_x_Bodyframe_UNIT_m_p_s2"
  Gain7/1 -> Bus Creator/8  "Acc_y_Bodyframe_UNIT_m_p_s2"
  Gain8/1 -> Bus Creator/9  "Acc_z_Bodyframe_UNIT_m_p_s2"
  Bus Selector/8 -> Gain7/1  "<acc_y>"
  Bus Selector/9 -> Gain8/1  "<acc_z>"
  Bus Selector/12 -> Gain11/1  "<Hz>"
  Bus Selector/13 -> Gain22/1  "<height_data_fusion>"
  Bus Creator/1 -> Imu_Data/1  "Imu_Data"
  Bus Selector/10 -> Gain9/1  "<Hx>"
  Bus Selector/11 -> Gain10/1  "<Hy>"
  Gain9/1 -> Bus Creator/10  "Mag_x_noUnit_int16"
  Gain10/1 -> Bus Creator/11  "Mag_y_noUnit_int16"
  Gain11/1 -> Bus Creator/12  "Mag_z_noUnit_int16"
  Gain22/1 -> Bus Creator/13  "Height_DataFusion_UNIT_m"
  Bus Selector/14 -> Gain23/1  "<dheight_data_fusion>"
  Gain23/1 -> Bus Creator/14  "Height_dot_DataFusion_UNIT_m_p_s"
  Bus Selector/15 -> Gain12/1  "<data_fusion_speed_EW>"
  Gain12/1 -> Bus Creator/15  "Speed_EW_DataFusion_UNIT_m_p_s"
  Bus Selector/16 -> Gain13/1  "<data_fusion_speed_NS>"
  Gain13/1 -> Bus Creator/16  "Speed_NS_DataFusion_UNIT_m_p_s"
  Bus Selector/17 -> Gain14/1  "<gps_latitude_data_fusion>"
  Gain14/1 -> Bus Creator/17  "Latitude_DataFusion_UNIT_deg"
  Bus Selector/18 -> Gain15/1  "<gps_longitude_data_fusion>"
  Gain15/1 -> Bus Creator/18  "Longitude_DataFusion_UNIT_deg"

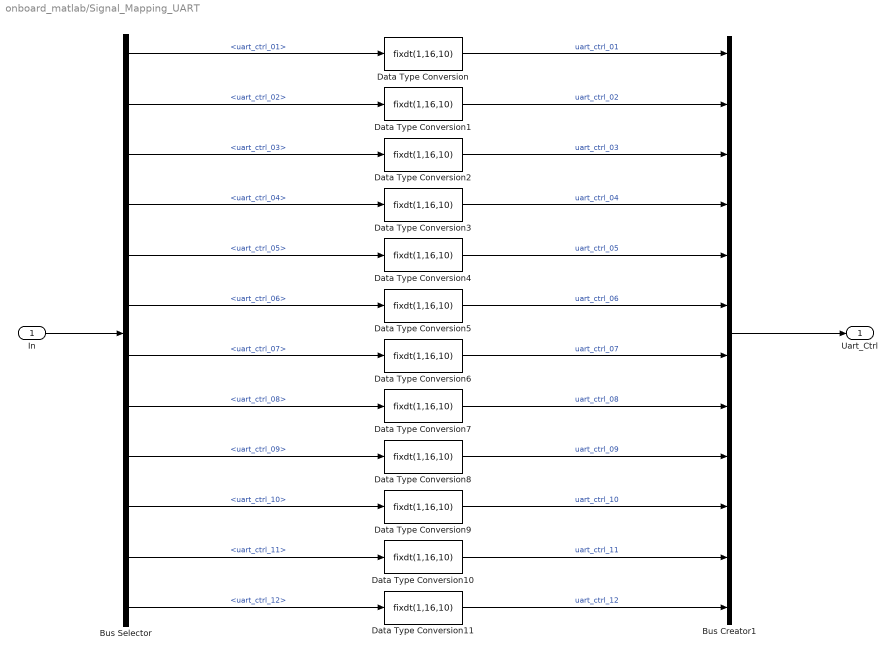
== system onboard_matlab/Signal_Mapping_UART ==
  In : Inport
  Bus Creator1 : BusCreator  Inputs=12
  Bus Selector : BusSelector  OutputSignals=uart_ctrl_01,uart_ctrl_02,uart_ctrl_03,uart_ctrl_04,uart_ctrl_05,uart_ctrl_06,uart_ctrl_07,uart_ctrl_08,uart_ctrl_09,uart_ctrl_10,uart_ctrl_11,uart_ctrl_12
  Data Type Conversion{,1..11} (12 alike) : DataTypeConversion  OutDataTypeStr=fixdt(1,16,10)  ConvertRealWorld=Stored Integer (SI)
  Uart_Ctrl : Outport
  wires:
  In/1 -> Bus Selector/1
  Bus Creator1/1 -> Uart_Ctrl/1
  Bus Selector/1 -> Data Type Conversion/1  "<uart_ctrl_01>"
  Bus Selector/2 -> Data Type Conversion1/1  "<uart_ctrl_02>"
  Bus Selector/3 -> Data Type Conversion2/1  "<uart_ctrl_03>"
  Bus Selector/4 -> Data Type Conversion3/1  "<uart_ctrl_04>"
  Bus Selector/5 -> Data Type Conversion4/1  "<uart_ctrl_05>"
  Bus Selector/6 -> Data Type Conversion5/1  "<uart_ctrl_06>"
  Bus Selector/7 -> Data Type Conversion6/1  "<uart_ctrl_07>"
  Bus Selector/8 -> Data Type Conversion7/1  "<uart_ctrl_08>"
  Bus Selector/9 -> Data Type Conversion8/1  "<uart_ctrl_09>"
  Bus Selector/10 -> Data Type Conversion9/1  "<uart_ctrl_10>"
  Data Type Conversion/1 -> Bus Creator1/1  "uart_ctrl_01"
  Data Type Conversion1/1 -> Bus Creator1/2  "uart_ctrl_02"
  Data Type Conversion2/1 -> Bus Creator1/3  "uart_ctrl_03"
  Data Type Conversion3/1 -> Bus Creator1/4  "uart_ctrl_04"
  Data Type Conversion4/1 -> Bus Creator1/5  "uart_ctrl_05"
  Data Type Conversion5/1 -> Bus Creator1/6  "uart_ctrl_06"
  Data Type Conversion6/1 -> Bus Creator1/7  "uart_ctrl_07"
  Data Type Conversion7/1 -> Bus Creator1/8  "uart_ctrl_08"
  Data Type Conversion8/1 -> Bus Creator1/9  "uart_ctrl_09"
  Data Type Conversion9/1 -> Bus Creator1/10  "uart_ctrl_10"
  Bus Selector/11 -> Data Type Conversion10/1  "<uart_ctrl_11>"
  Bus Selector/12 -> Data Type Conversion11/1  "<uart_ctrl_12>"
  Data Type Conversion10/1 -> Bus Creator1/11  "uart_ctrl_11"
  Data Type Conversion11/1 -> Bus Creator1/12  "uart_ctrl_12"

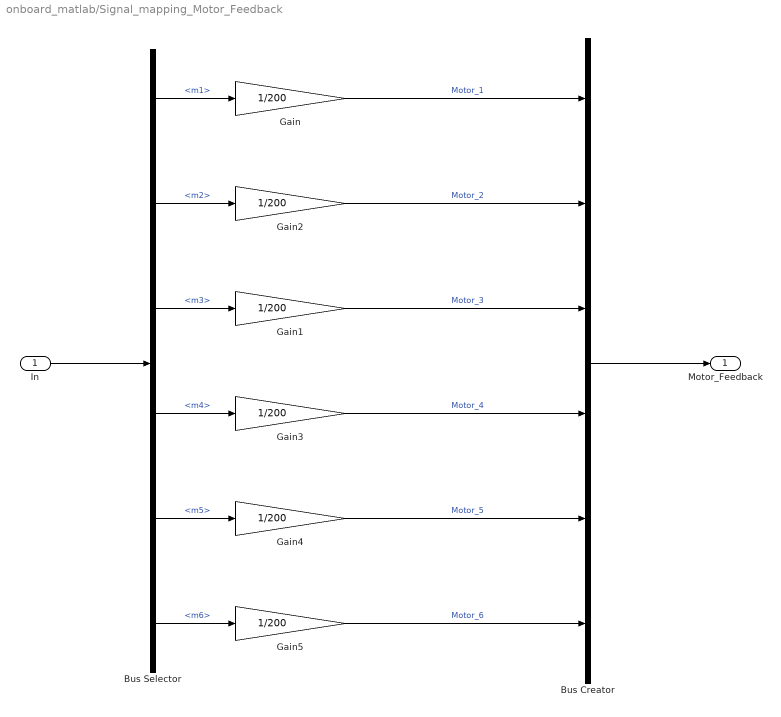
== system onboard_matlab/Signal_mapping_Motor_Feedback ==
  In : Inport
  Bus Creator : BusCreator  Inputs=6
  Bus Selector : BusSelector  OutputSignals=m1,m2,m3,m4,m5,m6
  Gain{,1..5} (6 alike) : Gain  Gain=1/200  OutMin=0  OutMax=1  OutDataTypeStr=fixdt(1,16,14)  RndMeth=Simplest  LockScale=on
  Motor_Feedback : Outport
  wires:
  In/1 -> Bus Selector/1
  Gain/1 -> Bus Creator/1  "Motor_1"
  Gain2/1 -> Bus Creator/2  "Motor_2"
  Gain1/1 -> Bus Creator/3  "Motor_3"
  Gain3/1 -> Bus Creator/4  "Motor_4"
  Gain4/1 -> Bus Creator/5  "Motor_5"
  Gain5/1 -> Bus Creator/6  "Motor_6"
  Bus Selector/1 -> Gain/1  "<m1>"
  Bus Selector/2 -> Gain2/1  "<m2>"
  Bus Selector/3 -> Gain1/1  "<m3>"
  Bus Selector/4 -> Gain3/1  "<m4>"
  Bus Selector/5 -> Gain4/1  "<m5>"
  Bus Selector/6 -> Gain5/1  "<m6>"
  Bus Creator/1 -> Motor_Feedback/1

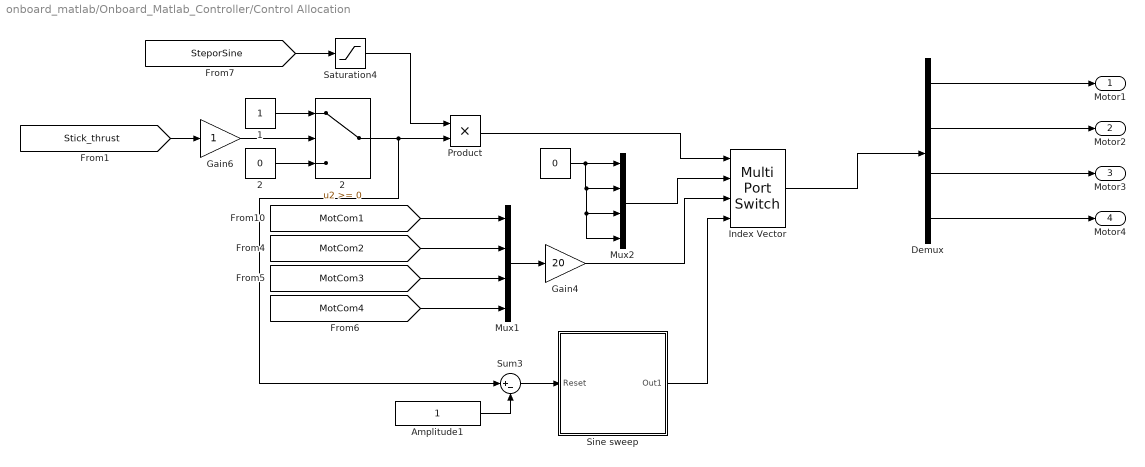
== system onboard_matlab/Onboard_Matlab_Controller/Control Allocation ==
  "   " : Constant  Value=0  OutDataTypeStr=fixdt(1,32,28)
  "   1" : Constant  OutDataTypeStr=fixdt(1,32,16)
  "   2" : Constant  Value=0  OutDataTypeStr=fixdt(1,32,16)
  " 2" : Switch  OutDataTypeStr=fixdt(1,32,16)
  Amplitude1 : Constant  OutMin=-2^15  OutMax=2^15-1  OutDataTypeStr=fixdt(1,32,16)
  Demux : Demux
  Gain4 : Gain  Gain=20  OutDataTypeStr=fixdt(1,32,16)  SaturateOnIntegerOverflow=on
  Gain6 : Gain  OutDataTypeStr=fixdt(1,32,16)  SaturateOnIntegerOverflow=on
  Index Vector : MultiPortSwitch  DataPortOrder=Zero-based contiguous  zeroidx=on
  Mux1 : Mux
  Mux2 : Mux
  Product : Product
  Saturation4 : Saturate  UpperLimit=2  LowerLimit=0  OutDataTypeStr=uint8  RndMeth=Zero
  Sine sweep : Subsystem
  Sum3 : Sum  Inputs=|+-  SaturateOnIntegerOverflow=on
  Motor1 : Outport
  Motor2 : Outport  Port=2
  Motor3 : Outport  Port=3
  Motor4 : Outport  Port=4
  wires:
  Demux/2 -> Motor2/1
  Demux/3 -> Motor3/1
  Demux/4 -> Motor4/1
  Demux/1 -> Motor1/1
  Sine sweep/1(Out1) -> Index Vector/4
  "   2"/1 -> " 2"/3
  [Stick_thrust] -> Gain6/1
  "   1"/1 -> " 2"/1
  Gain6/1 -> " 2"/2
  [SteporSine] -> Saturation4/1
  Saturation4/1 -> Product/1
  Mux2/1 -> Index Vector/2
  Mux1/1 -> Gain4/1
  [MotCom1] -> Mux1/1
  [MotCom2] -> Mux1/2
  [MotCom3] -> Mux1/3
  [MotCom4] -> Mux1/4
  Gain4/1 -> Index Vector/3
  Product/1 -> Index Vector/1
  "   "/1 -> Mux2/4, Mux2/3, Mux2/2, Mux2/1
  Index Vector/1 -> Demux/1
  " 2"/1 -> Sum3/1, Product/2
  Amplitude1/1 -> Sum3/2
  Sum3/1 -> Sine sweep/1(Reset)

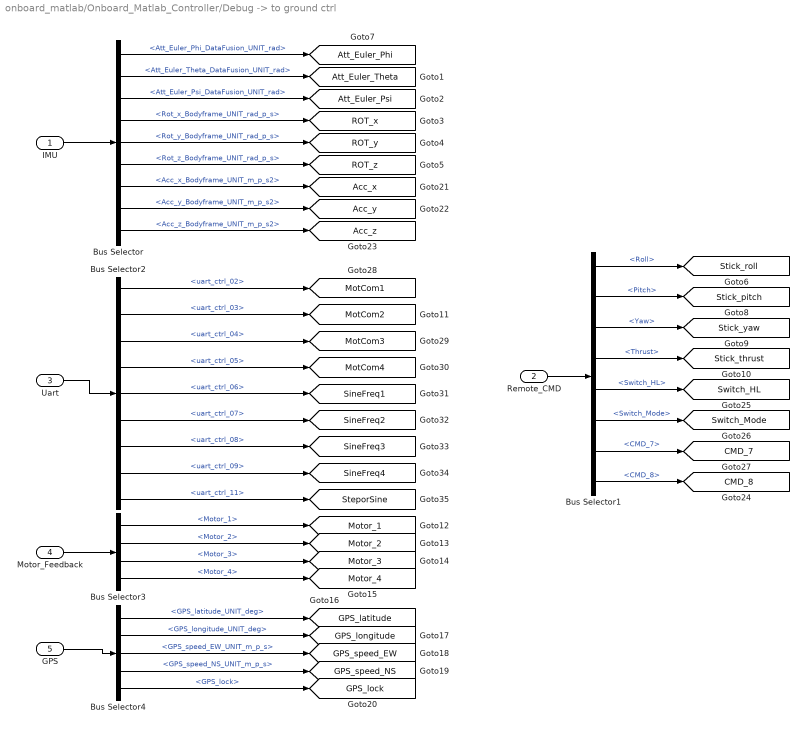
== system onboard_matlab/Onboard_Matlab_Controller/Debug -> to ground ctrl ==
  IMU : Inport
  Remote_CMD : Inport  Port=2
  Uart : Inport  Port=3
  Motor_Feedback : Inport  Port=4
  GPS : Inport  Port=5
  Bus Selector : BusSelector  OutputSignals=Att_Euler_Phi_DataFusion_UNIT_rad,Att_Euler_Theta_DataFusion_UNIT_rad,Att_Euler_Psi_DataFusion_UNIT_rad,Rot_x_Bodyframe_UNIT_rad_p_s,Rot_y_Bodyframe_UNIT_rad_p_s,Rot_z_Bodyframe_UNIT_rad_p_s,Acc_x_Bodyframe_UNIT_m_p_s2,Acc_y_Bodyframe_UNIT_m_p_s2,Acc_z_Bodyframe_UNIT_m_p_s2
  Bus Selector1 : BusSelector  OutputSignals=Roll,Pitch,Yaw,Thrust,Switch_HL,Switch_Mode,CMD_7,CMD_8
  Bus Selector2 : BusSelector  OutputSignals=uart_ctrl_02,uart_ctrl_03,uart_ctrl_04,uart_ctrl_05,uart_ctrl_06,uart_ctrl_07,uart_ctrl_08,uart_ctrl_09,uart_ctrl_11
  Bus Selector3 : BusSelector  OutputSignals=Motor_1,Motor_2,Motor_3,Motor_4
  Bus Selector4 : BusSelector  OutputSignals=GPS_latitude_UNIT_deg,GPS_longitude_UNIT_deg,GPS_speed_EW_UNIT_m_p_s,GPS_speed_NS_UNIT_m_p_s,GPS_lock
  tag scope: Acc_x=global, Acc_y=global, Acc_z=global, Att_Euler_Phi=global, Att_Euler_Psi=global, Att_Euler_Theta=global, CMD_7=global, CMD_8=global, GPS_latitude=global, GPS_lock=global, GPS_longitude=global, GPS_speed_EW=global, GPS_speed_NS=global, MotCom1=global, MotCom2=global, MotCom3=global, MotCom4=global, Motor_1=global, Motor_2=global, Motor_3=global, Motor_4=global, ROT_x=global, ROT_y=global, ROT_z=global, SineFreq1=global, SineFreq2=global, SineFreq3=global, SineFreq4=global, SteporSine=global, Stick_pitch=global, Stick_roll=global, Stick_thrust=global, Stick_yaw=global, Switch_HL=global, Switch_Mode=global
  wires:
  IMU/1 -> Bus Selector/1
  Bus Selector/1 -> [Att_Euler_Phi]  "<Att_Euler_Phi_DataFusion_UNIT_rad>"
  Bus Selector/2 -> [Att_Euler_Theta]  "<Att_Euler_Theta_DataFusion_UNIT_rad>"
  Bus Selector/3 -> [Att_Euler_Psi]  "<Att_Euler_Psi_DataFusion_UNIT_rad>"
  Bus Selector/4 -> [ROT_x]  "<Rot_x_Bodyframe_UNIT_rad_p_s>"
  Bus Selector/5 -> [ROT_y]  "<Rot_y_Bodyframe_UNIT_rad_p_s>"
  Bus Selector/6 -> [ROT_z]  "<Rot_z_Bodyframe_UNIT_rad_p_s>"
  Remote_CMD/1 -> Bus Selector1/1
  Bus Selector1/1 -> [Stick_roll]  "<Roll>"
  Bus Selector1/2 -> [Stick_pitch]  "<Pitch>"
  Bus Selector1/3 -> [Stick_yaw]  "<Yaw>"
  Bus Selector1/4 -> [Stick_thrust]  "<Thrust>"
  Uart/1 -> Bus Selector2/1
  Motor_Feedback/1 -> Bus Selector3/1
  Bus Selector3/1 -> [Motor_1]  "<Motor_1>"
  Bus Selector3/2 -> [Motor_2]  "<Motor_2>"
  Bus Selector3/3 -> [Motor_3]  "<Motor_3>"
  Bus Selector3/4 -> [Motor_4]  "<Motor_4>"
  GPS/1 -> Bus Selector4/1
  Bus Selector4/1 -> [GPS_latitude]  "<GPS_latitude_UNIT_deg>"
  Bus Selector4/2 -> [GPS_longitude]  "<GPS_longitude_UNIT_deg>"
  Bus Selector4/3 -> [GPS_speed_EW]  "<GPS_speed_EW_UNIT_m_p_s>"
  Bus Selector4/4 -> [GPS_speed_NS]  "<GPS_speed_NS_UNIT_m_p_s>"
  Bus Selector4/5 -> [GPS_lock]  "<GPS_lock>"
  Bus Selector/7 -> [Acc_x]  "<Acc_x_Bodyframe_UNIT_m_p_s2>"
  Bus Selector/8 -> [Acc_y]  "<Acc_y_Bodyframe_UNIT_m_p_s2>"
  Bus Selector/9 -> [Acc_z]  "<Acc_z_Bodyframe_UNIT_m_p_s2>"
  Bus Selector1/5 -> [Switch_HL]  "<Switch_HL>"
  Bus Selector1/6 -> [Switch_Mode]  "<Switch_Mode>"
  Bus Selector1/7 -> [CMD_7]  "<CMD_7>"
  Bus Selector1/8 -> [CMD_8]  "<CMD_8>"
  Bus Selector2/1 -> [MotCom1]  "<uart_ctrl_02>"
  Bus Selector2/2 -> [MotCom2]  "<uart_ctrl_03>"
  Bus Selector2/3 -> [MotCom3]  "<uart_ctrl_04>"
  Bus Selector2/4 -> [MotCom4]  "<uart_ctrl_05>"
  Bus Selector2/5 -> [SineFreq1]  "<uart_ctrl_06>"
  Bus Selector2/6 -> [SineFreq2]  "<uart_ctrl_07>"
  Bus Selector2/7 -> [SineFreq3]  "<uart_ctrl_08>"
  Bus Selector2/8 -> [SineFreq4]  "<uart_ctrl_09>"
  Bus Selector2/9 -> [SteporSine]  "<uart_ctrl_11>"

== system onboard_matlab/Output_Mapping_Debug/List_Iterator ==
  Constant1 : Constant  OutDataTypeStr=int16
  Constant2 : Constant  OutDataTypeStr=int16
  Constant3 : Constant  Value=dec  OutMin=1  OutDataTypeStr=int16
  Constant4 : Constant  Value=list  OutDataTypeStr=int16
  Divide : Product  Inputs=*/  OutDataTypeStr=int16  RndMeth=Ceiling  InputSameDT=on
  FixPt Switch : Switch  Criteria=u2 > Threshold  Threshold=length(list)*dec  OutDataTypeStr=Inherit: Inherit via back propagation  ZeroCross=off  InputSameDT=on
  Index Vector : MultiPortSwitch  Inputs=1
  Sum : Sum  Inputs=++|  AccumDataTypeStr=int16  OutDataTypeStr=int16
  Unit Delay : UnitDelay  InitialCondition=1  SampleTime=-1
  index : Outport
  wires:
  Divide/1 -> Index Vector/1
  Index Vector/1 -> index/1
  Constant4/1 -> Index Vector/2
  Constant3/1 -> Divide/2
  Constant2/1 -> Sum/2
  Constant1/1 -> FixPt Switch/1
  Sum/1 -> FixPt Switch/2, FixPt Switch/3
  FixPt Switch/1 -> Unit Delay/1
  Unit Delay/1 -> Divide/1, Sum/1

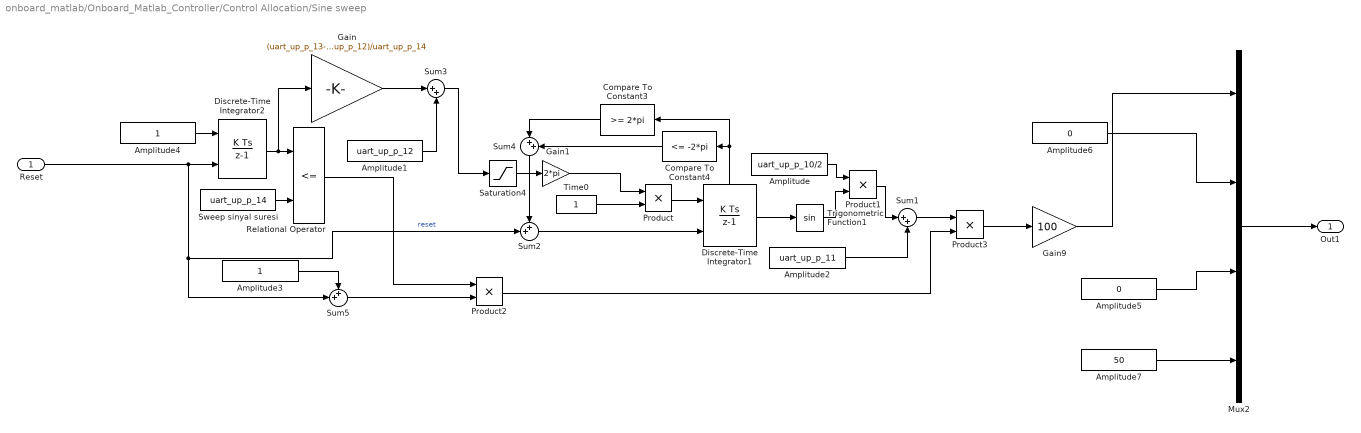
== system onboard_matlab/Onboard_Matlab_Controller/Control Allocation/Sine sweep ==
  Reset : Inport
  Amplitude : Constant  Value=uart_up_p_10/2  OutMin=-2^15  OutMax=2^15-1  OutDataTypeStr=fixdt(1,32,16)
  Amplitude1 : Constant  Value=uart_up_p_12  OutMin=-2^15  OutMax=2^15-1  OutDataTypeStr=fixdt(1,32,16)
  Amplitude2 : Constant  Value=uart_up_p_11  OutMin=-2^15  OutMax=2^15-1  OutDataTypeStr=fixdt(1,32,16)
  Amplitude3 : Constant  OutMin=-2^15  OutMax=2^15-1  OutDataTypeStr=fixdt(1,32,16)
  Amplitude4 : Constant  OutMin=-2^15  OutMax=2^15-1  OutDataTypeStr=fixdt(1,32,16)
  Amplitude5 : Constant  Value=0  OutMin=-2^15  OutMax=2^15-1  OutDataTypeStr=fixdt(1,32,16)
  Amplitude6 : Constant  Value=0  OutMin=-2^15  OutMax=2^15-1  OutDataTypeStr=fixdt(1,32,16)
  Amplitude7 : Constant  Value=50  OutMin=-2^15  OutMax=2^15-1  OutDataTypeStr=fixdt(1,32,16)
  Compare To Constant3 : simulink/Logic and Bit Operations/Compare To Constant  relop=>=  const=2*pi  OutDataTypeStr=uint8  ZeroCross=off
  Compare To Constant4 : simulink/Logic and Bit Operations/Compare To Constant  relop=<=  const=-2*pi  OutDataTypeStr=uint8  ZeroCross=off
  Discrete-Time Integrator1 : DiscreteIntegrator  ExternalReset=level  InitialConditionMode=State only (most efficient)  SampleTime=-1  OutMax=2*pi  OutDataTypeStr=fixdt(1,32,28)  RndMeth=Zero  LimitOutput=on  UpperSaturationLimit=2*pi  LowerSaturationLimit=-2*pi  ShowStatePort=on  ICPrevOutput=DiscIntNeverNeededParam  ICPrevScaledInput=DiscIntNeverNeededParam
  Discrete-Time Integrator2 : DiscreteIntegrator  ExternalReset=level  InitialConditionMode=State only (most efficient)  SampleTime=-1  OutDataTypeStr=fixdt(1,32,21)  RndMeth=Zero  UpperSaturationLimit=2*pi  LowerSaturationLimit=-2*pi  ICPrevOutput=DiscIntNeverNeededParam  ICPrevScaledInput=DiscIntNeverNeededParam
  Gain : Gain  Gain=(uart_up_p_13-uart_up_p_12)/uart_up_p_14
  Gain1 : Gain  Gain=2*pi
  Gain9 : Gain  Gain=100  OutDataTypeStr=fixdt(1,32,16)
  Mux2 : Mux
  Product{,1..3} (4 alike) : Product
  Relational Operator : RelationalOperator  Operator=<=  OutDataTypeStr=fixdt(1,16)
  Saturation4 : Saturate  UpperLimit=32  LowerLimit=0  OutDataTypeStr=fixdt(1,16,10)  RndMeth=Zero
  Sum1 : Sum  Inputs=|++  SaturateOnIntegerOverflow=on
  Sum2 : Sum  Inputs=++|  AccumDataTypeStr=int8  OutDataTypeStr=int8  SaturateOnIntegerOverflow=on
  Sum3 : Sum  Inputs=|++  SaturateOnIntegerOverflow=on
  Sum4 : Sum  Inputs=|++  AccumDataTypeStr=int8  OutDataTypeStr=int8  SaturateOnIntegerOverflow=on
  Sum5 : Sum  Inputs=++|  SaturateOnIntegerOverflow=on
  Sweep sinyal suresi : Constant  Value=uart_up_p_14  OutMin=-2^15  OutMax=2^15-1  OutDataTypeStr=fixdt(1,32,16)
  Time0 : Constant  OutDataTypeStr=fixdt(1,32,8)
  Trigonometric Function1 : Trigonometry  ApproximationMethod=CORDIC
  Out1 : Outport
  wires:
  Reset/1 -> Sum5/2, Sum2/2, Discrete-Time Integrator2/2  "reset"
  Amplitude1/1 -> Sum3/2
  Amplitude4/1 -> Discrete-Time Integrator2/1
  Sweep sinyal suresi/1 -> Relational Operator/2
  Discrete-Time Integrator2/1 -> Relational Operator/1, Gain/1
  Gain/1 -> Sum3/1
  Compare To Constant4/1 -> Sum4/2
  Compare To Constant3/1 -> Sum4/1
  Sum4/1 -> Sum2/1
  Discrete-Time Integrator1/State -> Compare To Constant3/1, Compare To Constant4/1
  Saturation4/1 -> Gain1/1
  Time0/1 -> Product/2
  Product/1 -> Discrete-Time Integrator1/1
  Discrete-Time Integrator1/1 -> Trigonometric Function1/1
  Amplitude2/1 -> Sum1/2
  Trigonometric Function1/1 -> Product1/2
  Product1/1 -> Sum1/1
  Sum3/1 -> Saturation4/1
  Gain1/1 -> Product/1
  Sum2/1 -> Discrete-Time Integrator1/2
  Amplitude/1 -> Product1/1
  Sum1/1 -> Product3/1
  Product3/1 -> Gain9/1
  Gain9/1 -> Mux2/1
  Relational Operator/1 -> Product2/1
  Sum5/1 -> Product2/2
  Product2/1 -> Product3/2
  Amplitude3/1 -> Sum5/1
  Mux2/1 -> Out1/1
  Amplitude5/1 -> Mux2/3
  Amplitude7/1 -> Mux2/4
  Amplitude6/1 -> Mux2/2
